simulink model "Torque Vectoring and Ackerman Model"  (R2020b)
settings: Solver=ode4  StartTime=0.0  StopTime=12  FixedStep=1e-5  RelTol=1e-3
InitFcn:
  | clc
  | clear
  | clc;
  | clear;
  | Ts=1e-5; %Sampling time
  | f=50; %Supply frequency
  | Rs=0.03553; %Stator resistance
  | Rr=0.02092; %Rotor resistance
  | Lls=0.000335; %Stator inductance
  | Llr=0.000335; %Rotor inductance
  | Lm=0.0151; %Mutual inductance
  | P=4; %Number of Poles
  | ts=(Lls+Lm)/Rs; % Stator time constant
  | Tr=(Llr+Lm)/Rr; % Rotor time constant
  | Ls=Lls+Lm;
  | Lrr=Llr+Lm;
  | J=1.25; %Inertia
  | F=0.03914; %Friction factor
  | VDC=580;
  | sigma=1-(Lm^2/(Ls*Lrr));
  | rs=Rs+Rr*(Lm/Lrr)^2;
  | Kp=1498*sigma*Ls;
  | Ki=rs*1498;
  | dw=1.55;
  | l=3;
  | m       =       1500;           %Vehicle mass
  | g       =       9.81;           %Gravitational acceleration
  | L       =          3;           %Distance between front axle and rear axle
  | Lf      =        1.3;           %Distance between center of mass and front axle
  | Lr      =       L-Lf;           %Distance between center of mass and rear axle
  | Cf      =      67369;           %Front track Cornering stiffness coef
  | Cr      =      63411;           %rear track Cornering stiffness coef
  | S       =        1.7;           %Area of frontal surface of the vehicle
  | CYB     =       -2.2;           %Force drag coef
  | CMzB    =        0.6;           %Moment drag coef
  | Mzfa    =       2010;           %Front track Aligning stiffness coef
  | Mzra    =       1366;           %rear track Aligning stiffness coef
  | rho     =      1.225;           %density
  | Iz      =       2000;           %Yaw Moment of Inertia
  | Kgear=1;
undefined symbols (not defined in the file): DiscIntNeverNeededParam, Driver, Wheels_Driver_VehDyn_Lib
libraries: pid_lib x12, powerlib_meascontrol x11, powerlib x9, simulink_extras x4
(part 1 of 2)
settings Model: Creator=Mostafa  LastModifiedBy=Mostafa

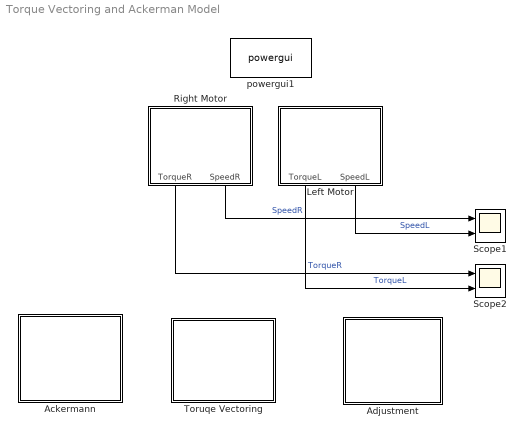
== system Torque Vectoring and Ackerman Model ==
  Ackermann : Subsystem
  Adjustment : Subsystem
  Left Motor : Subsystem
      settings: PortSchema="{\"entries\":[{\"content\":{\"sides\":[{\"content\":{\"connectorIds\":[]},\"type\":\"ConnectorPlacement.EquallySpacedRectSide\",\"uuid\":\"d60caa5e-c143-44b9-abe1-e5bc42f5c989\"},{\"content\":{\"connectorIds\":[],\"side\":\"RIGHT\"},\"type\":\"ConnectorPlacement.EquallySpacedRectSide\",\"uuid\":\"6d3ab839-fc24-43f3-9ba9-29c9b61bd22e\"},{\"content\":{\"connectorIds\":[],\"side\":\"TOP\"},\"type\":\"ConnectorPlacement.EquallySpacedRectSide\",\"uuid\":\"19f78343-3a34-4d8d-b4ff-ce8c56708ba0\"},{\"content\":{\"connectorIds\":[\"Out1\",\"Out2\"],\"side\":\"BOTTOM\"},\"type\":\"ConnectorPlacement.EquallySpacedRectSide\",\"uuid\":\"b455b762-473b-46a0-b917-5ab7203214ed\"},{\"content\":{\"connectorIds\":[],\"side\":\"HIDDEN\"},\"type\":\"ConnectorPlacement.EquallySpacedRectSide\",\"uuid\":\"ac9f86ca-680b-4222-bdb6-29216a90dea9\"}]},\"type\":\"ConnectorPlacement.EquallySpacedConnector\",\"uuid\":\"3823dedf-6920-4310-aeb6-55963e7ef5a8\"}],\"packageUris\":[\"http://schema.mathworks.com/mf0/Connector/R2020b\"],\"version\":\"1.0\"}"
      mask Display: image('D:\images.jpg'); % Use "Edit Image" on toolstrip to change.
  Right Motor : Subsystem
      settings: PortSchema="{\"entries\":[{\"content\":{\"sides\":[{\"content\":{\"connectorIds\":[]},\"type\":\"ConnectorPlacement.EquallySpacedRectSide\",\"uuid\":\"d60caa5e-c143-44b9-abe1-e5bc42f5c989\"},{\"content\":{\"connectorIds\":[],\"side\":\"RIGHT\"},\"type\":\"ConnectorPlacement.EquallySpacedRectSide\",\"uuid\":\"6d3ab839-fc24-43f3-9ba9-29c9b61bd22e\"},{\"content\":{\"connectorIds\":[],\"side\":\"TOP\"},\"type\":\"ConnectorPlacement.EquallySpacedRectSide\",\"uuid\":\"19f78343-3a34-4d8d-b4ff-ce8c56708ba0\"},{\"content\":{\"connectorIds\":[\"Out1\",\"Out2\"],\"side\":\"BOTTOM\"},\"type\":\"ConnectorPlacement.EquallySpacedRectSide\",\"uuid\":\"35fd2daf-de54-41dc-b20d-56980127e7c6\"},{\"content\":{\"connectorIds\":[],\"side\":\"HIDDEN\"},\"type\":\"ConnectorPlacement.EquallySpacedRectSide\",\"uuid\":\"ac9f86ca-680b-4222-bdb6-29216a90dea9\"}]},\"type\":\"ConnectorPlacement.EquallySpacedConnector\",\"uuid\":\"3823dedf-6920-4310-aeb6-55963e7ef5a8\"}],\"packageUris\":[\"http://schema.mathworks.com/mf0/Connector/R2020b\"],\"version\":\"1.0\"}"
      mask Display: image('D:\images.jpg'); % Use "Edit Image" on toolstrip to change.
  Scope1 : Scope  NumInputPorts=2
  Scope2 : Scope  NumInputPorts=2
  Toruqe Vectoring : Subsystem
  powergui1 : powerlib/powergui  Priority=1  SimulationMode=Continuous  SampleTime=1e-6  frequency=60  Iterations=50  frequencyindice=50  Pbase=100e6  ErrMax=1e-4  UnitsV=kV  UnitsW=MW  buscounter=0  FunctionMessages=off  echomessages=off  EnableUseOfTLC=off  CurrentSourceSwitches=off  DisableSnubberDevices=off  DisableRonSwitches=off  DisableVfSwitches=off  DisplayEquations=off  AutomaticDiscreteSolvers=off  SolverType=Tustin/Backward Euler (TBE)  Interpol=off  ExternalGateDelay=off  methode=off  Ts=100  x0status=blocks  SPID=on  SwTol=0  HookPort=off  NonlinearTolerance=1e-4  nMaxIteration=100  ContinueOnMaxIteration=off  RestoreLinks=warning  ResistiveCurrentMeasurement=off  Frange=[0:2:500]  Ylog=off  Xlog=on  ShowGrid=off  save=off  variable=ZData  structure=0  ZoomFFT=off  StartTime=0.0  cycles=1  DisplayStyle=1  fundamental=60  FreqAxis=off  MaxFrequency=1000  frequencyindicesteady=1  RmsSteady=1  display=off
  wires:
  Right Motor/2(SpeedR) -> Scope1/1  "SpeedR"
  Left Motor/2(SpeedL) -> Scope1/2  "SpeedL"
  Right Motor/1(TorqueR) -> Scope2/1  "TorqueR"
  Left Motor/1("TorqueL ") -> Scope2/2  "TorqueL"

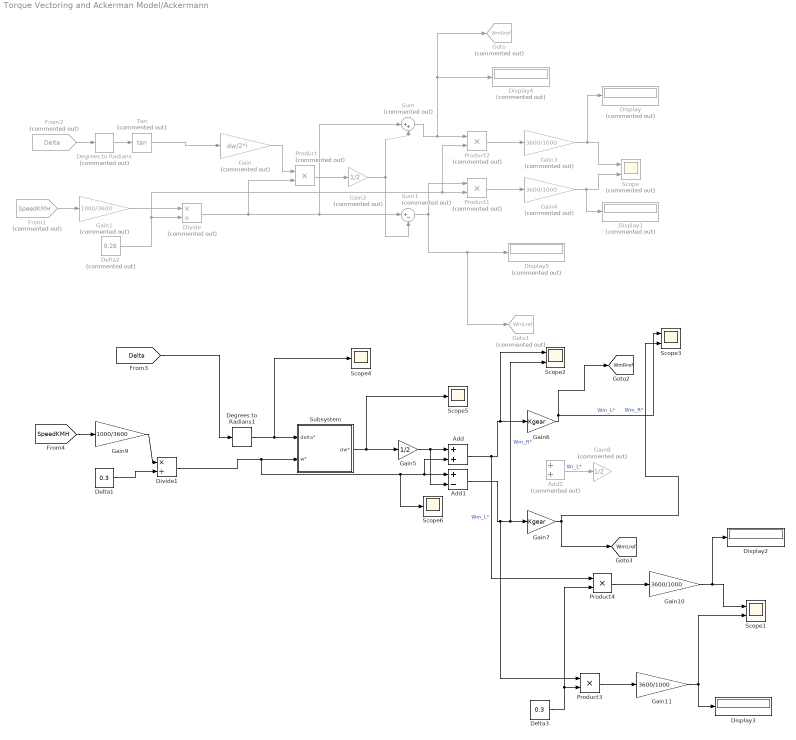
== system Torque Vectoring and Ackerman Model/Ackermann ==
  Add : Sum
  Add1 : Sum  Inputs=+-
  Add2 : Sum  Commented=on
  Degrees to Radians : simulink_extras/Transformations/Degrees to Radians  Commented=on
  Degrees to Radians1 : simulink_extras/Transformations/Degrees to Radians
  Delta1 : Constant  Value=0.3
  Delta2 : Constant  Commented=on  Value=0.26
  Delta3 : Constant  Value=0.3
  Display{,1,4..5} (4 alike) : Display  Commented=on
  Display2 : Display
  Display3 : Display
  Divide : Product  Commented=on  Inputs=*/
  Divide1 : Product  Inputs=*/
  From1 : From  Commented=on  GotoTag=SpeedKMH  TagVisibility=global
  From2 : From  Commented=on  GotoTag=Delta  TagVisibility=global
  Gain : Gain  Commented=on  Gain=dw/2*l
  Gain1 : Gain  Commented=on  Gain=1000/3600
  Gain10 : Gain  Gain=3600/1000
  Gain11 : Gain  Gain=3600/1000
  Gain2 : Gain  Commented=on  Gain=1/2
  Gain3 : Gain  Commented=on  Gain=3600/1000
  Gain4 : Gain  Commented=on  Gain=3600/1000
  Gain5 : Gain  Gain=1/2
  Gain6 : Gain  Gain=Kgear
  Gain7 : Gain  Gain=Kgear
  Gain8 : Gain  Commented=on  Gain=1/2
  Gain9 : Gain  Gain=1000/3600
  Goto : Goto  Commented=on  GotoTag=WmRref  TagVisibility=global
  Goto1 : Goto  Commented=on  GotoTag=WmLref  TagVisibility=global
  Product : Product  Commented=on
  Product1 : Product  Commented=on
  Product2 : Product  Commented=on
  Product3 : Product
  Product4 : Product
  Scope : Scope  Commented=on  NumInputPorts=2
  Scope1 : Scope  NumInputPorts=2
  Scope2 : Scope  NumInputPorts=2
  Scope3 : Scope  NumInputPorts=2
  Scope4 : Scope
  Scope5 : Scope
  Scope6 : Scope
  Subsystem : Subsystem
  Sum : Sum  Commented=on  Inputs=|++
  Sum1 : Sum  Commented=on  Inputs=|+-
  Tan : Trigonometry  Commented=on  Operator=tan
  tag scope: WmLref=global, WmRref=global
  wires:
  Degrees to Radians/1 -> Tan/1
  Tan/1 -> Gain/1
  Gain/1 -> Product/1
  Product/1 -> Gain2/1
  Gain2/1 -> Sum1/2, Sum/2
  Divide/1 -> Product/2, Sum/1, Sum1/1
  Gain1/1 -> Divide/1
  Sum1/1 -> Product1/1, Goto1/1, Display5/1
  Delta2/1 -> Product2/2, Product1/2, Divide/2
  Product2/1 -> Gain3/1
  Product1/1 -> Gain4/1
  Gain4/1 -> Display1/1, Scope/2
  Gain3/1 -> Display/1, Scope/1
  Sum/1 -> Display4/1, Goto/1, Product2/1
  From1/1 -> Gain1/1
  From2/1 -> Degrees to Radians/1
  Degrees to Radians1/1 -> Scope4/1, Subsystem/1(delta*)
  Gain5/1 -> Add1/2, Add/1
  Gain6/1 -> Scope3/1, [WmRref]  "Wm_L*"
  Subsystem/1(dw*) -> Scope5/1, Gain5/1
  Add2/1 -> Gain8/1  "Wr_L*"
  Gain7/1 -> Scope3/2, [WmLref]  "Wm_R*"
  Gain9/1 -> Divide1/1
  [SpeedKMH] -> Gain9/1
  Delta1/1 -> Divide1/2
  [Delta] -> Degrees to Radians1/1
  Divide1/1 -> Scope6/1, Add/2, Add1/1, Subsystem/2(w*)
  Delta3/1 -> Product4/2, Product3/2
  Gain10/1 -> Scope1/1, Display2/1
  Product4/1 -> Gain10/1
  Gain11/1 -> Scope1/2, Display3/1
  Add/1 -> Product4/1, Scope2/1, Gain6/1  "Wm_L*"
  Add1/1 -> Product3/1, Scope2/2, Gain7/1  "Wm_R*"
  Product3/1 -> Gain11/1

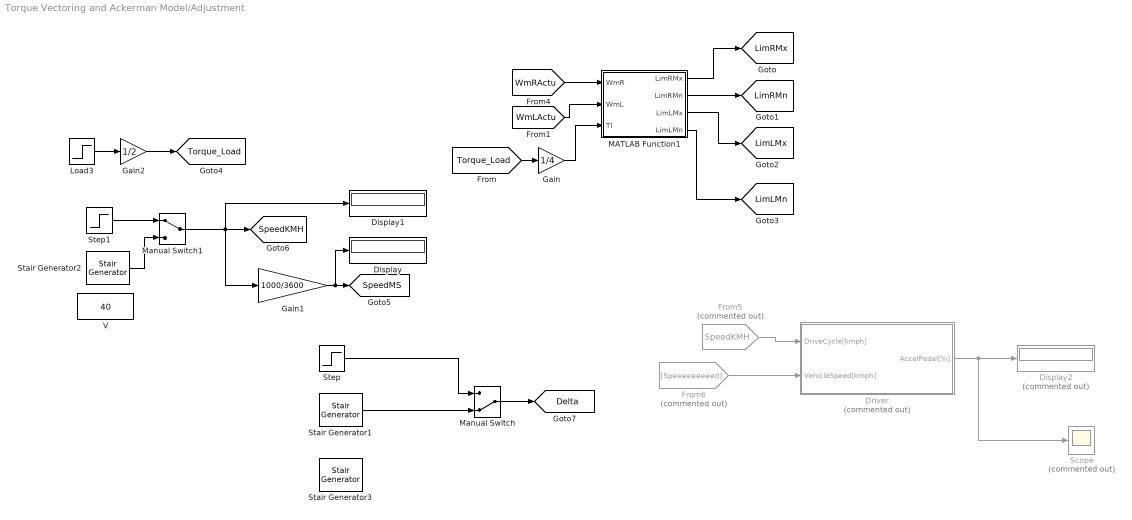
== system Torque Vectoring and Ackerman Model/Adjustment ==
  Display : Display
  Display1 : Display
  Display2 : Display  Commented=on
  Driver : Subsystem  Commented=on  AncestorBlock=Wheels_Driver_VehDyn_Lib/Driver
  From5 : From  Commented=on  GotoTag=SpeedKMH  TagVisibility=global
  From6 : From  Commented=on  GotoTag=Speeeeeeeeed  TagVisibility=global
  Gain : Gain  Gain=1/4
  Gain1 : Gain  Gain=1000/3600
  Gain2 : Gain  Gain=1/2
  Load3 : Step  Time=3  After=800  SampleTime=Ts
  MATLAB Function1 : MATLAB Function  TreatAsAtomicUnit=on
  Manual Switch : ManualSwitch  CurrentSetting=0
  Manual Switch1 : ManualSwitch
  Scope : Scope  Commented=on
  Stair Generator1 : powerlib_meascontrol/Pulse & Signal Generators/Stair Generator  t="[0 4 6 8 10  ]"  e=[0 10 0 -10 0 ]  Ts=0
  Stair Generator2 : powerlib_meascontrol/Pulse & Signal Generators/Stair Generator  t=[0 3 5 7 9 10 ]  e=[0 50 100 -50 -100 0 ]  Ts=0
  Stair Generator3 : powerlib_meascontrol/Pulse & Signal Generators/Stair Generator  t=[0 3 5 7 9 10 ]  e=[0 5 10 -5 10 0 ]  Ts=0
  Step : Step  Time=4  After=10  SampleTime=0
  Step1 : Step  Time=3  After=36  SampleTime=0
  V : Constant  Value=40
  tag scope: Delta=global, LimLMn=global, LimLMx=global, LimRMn=global, LimRMx=global, SpeedKMH=global, SpeedMS=global, Torque_Load=global
  wires:
  Gain1/1 -> Display/1, [SpeedMS]
  Load3/1 -> Gain2/1
  Step/1 -> Manual Switch/1
  Manual Switch/1 -> [Delta]
  Stair Generator1/1 -> Manual Switch/2
  [WmRActu] -> MATLAB Function1/1(WmR)
  [WmLActu] -> MATLAB Function1/2(WmL)
  MATLAB Function1/3(LimLMx) -> [LimLMx]
  MATLAB Function1/4(LimLMn) -> [LimLMn]
  MATLAB Function1/1(LimRMx) -> [LimRMx]
  MATLAB Function1/2(LimRMn) -> [LimRMn]
  Manual Switch1/1 -> Gain1/1, Display1/1, [SpeedKMH]
  Step1/1 -> Manual Switch1/1
  Stair Generator2/1 -> Manual Switch1/2
  [Torque_Load] -> Gain/1
  Gain/1 -> MATLAB Function1/3(Tl)
  From5/1 -> Driver/1(" DriveCycle[kmph]")
  From6/1 -> Driver/2(VehicleSpeed[kmph])
  Driver/1(AccelPedal[%]) -> Scope/1, Display2/1
  Gain2/1 -> [Torque_Load]

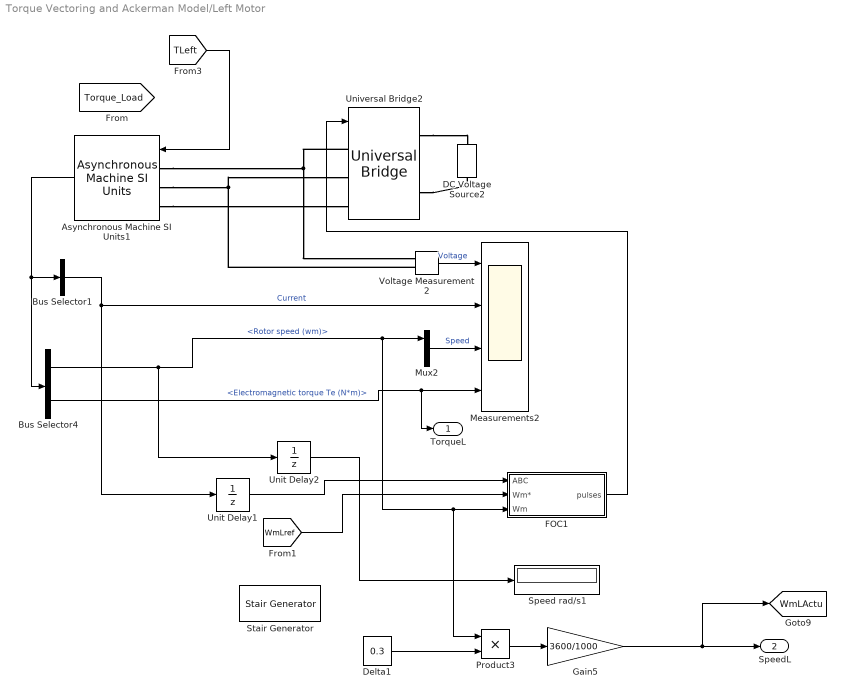
== system Torque Vectoring and Ackerman Model/Left Motor ==
  Asynchronous Machine SI Units1 : powerlib/Machines/Asynchronous Machine SI Units  RotorType=Squirrel-cage  PresetModel="19:  100 HP (75KW)  400 V 50Hz 1484 RPM"  MechanicalLoad=Torque Tm  ShowDetailedParameters=on  ReferenceFrame=Rotor  Units=SI  MeasurementBus=off  NominalParameters=[7.5e+04 400 50]  Stator=[0.03552 0.000335]  Rotor=[0.02092 0.000335]  Cage1=[0.4155 0.002066]  Cage2=[0.4168 0.0003495]  Lm=0.0151  Mechanical=[1.25 0.03914 2]  PolePairs=2  InitialConditions=[1 0 0 0 0 0 0 0]  SimulateSaturation=off  Saturation=[14.03593122, 27.81365428, 53.79336849, 72.68890987, 97.98006896, 148.6815601, 215.7428561, 302.9841135, 428.7778367 ; 230, 322, 414, 460, 506, 552, 598, 644, 690]  LoadFlowParameters=1492000  TsPowergui=0  TsBlock=-1  IterativeModel=Trapezoidal non iterative  IterativeDiscreteModel=Trapezoidal non iterative  Pmec=1.492e+006
  Bus Selector1 : BusSelector  OutputSignals=Stator measurements.Stator current is_a (A),Stator measurements.Stator current is_b (A),Stator measurements.Stator current is_c (A)  OutputAsBus=on
  Bus Selector4 : BusSelector  OutputSignals=Mechanical.Rotor speed (wm),Mechanical.Electromagnetic torque Te (N*m)
  DC Voltage Source2 : powerlib/Electrical Sources/DC Voltage Source  Amplitude=VDC  Measurements=None
  Delta1 : Constant  Value=0.3
  FOC1 : Subsystem
  Gain5 : Gain  Gain=3600/1000
  Measurements2 : Scope  NumInputPorts=4
  Mux2 : Mux  Inputs=2
  Product3 : Product
  Speed rad/s1 : Display
  Stair Generator : powerlib_meascontrol/Pulse & Signal Generators/Stair Generator  t=[0 2 3 4 5 6 ]  e=[0 95 60 105 70 -120 ]  Ts=Ts
  Unit Delay1 : UnitDelay  SampleTime=-1  HasFrameUpgradeWarning=on
  Unit Delay2 : UnitDelay  SampleTime=-1  HasFrameUpgradeWarning=on
  Universal Bridge2 : powerlib/Power Electronics/Universal Bridge  Arms=3  SnubberResistance=1e5  SnubberCapacitance=inf  Device=IGBT / Diodes  Ron=1e-3  Lon=0  ForwardVoltages="[  0  0  ]"  ForwardVoltage=0  GTOparameters=[ 10e-6 , 20e-6 ]  IGBTparameters=[ 1e-6 , 2e-6 ]  Measurements=None  Measurements_2=None  converterType=Rectifier
  Voltage Measurement2 : powerlib/Measurements/Voltage Measurement  PhasorSimulation=off  OutputType=Complex  PSBequivalent=0
  "TorqueL " : Outport
  SpeedL : Outport  Port=2
  tag scope: WmLActu=global
  wires:
  Voltage Measurement2/1 -> Measurements2/1  "Voltage"
  Asynchronous Machine SI Units1/1 -> Bus Selector1/1, Bus Selector4/1
  Bus Selector1/1 -> Measurements2/2, Unit Delay1/1  "Current"
  Bus Selector4/1 -> Unit Delay2/1, Mux2/1, Product3/1, FOC1/3(Wm)  "<Rotor speed (wm)>"
  Unit Delay2/1 -> Speed rad/s1/1
  Bus Selector4/2 -> "TorqueL "/1, Measurements2/4  "<Electromagnetic torque Te (N*m)>"
  Mux2/1 -> Measurements2/3  "Speed"
  Unit Delay1/1 -> FOC1/1(ABC)
  FOC1/1(pulses) -> Universal Bridge2/1
  Delta1/1 -> Product3/2
  Product3/1 -> Gain5/1
  [WmLref] -> FOC1/2(Wm*)
  [TLeft] -> Asynchronous Machine SI Units1/1
  Gain5/1 -> [WmLActu], SpeedL/1
  connections:
  Universal Bridge2/RConn2 -- DC Voltage Source2/LConn1
  Universal Bridge2/RConn1 -- DC Voltage Source2/RConn1
  Asynchronous Machine SI Units1/LConn3 -- Universal Bridge2/LConn3
  Voltage Measurement2/LConn2 -- Universal Bridge2/LConn2 -- Asynchronous Machine SI Units1/LConn2
  Universal Bridge2/LConn1 -- Voltage Measurement2/LConn1 -- Asynchronous Machine SI Units1/LConn1

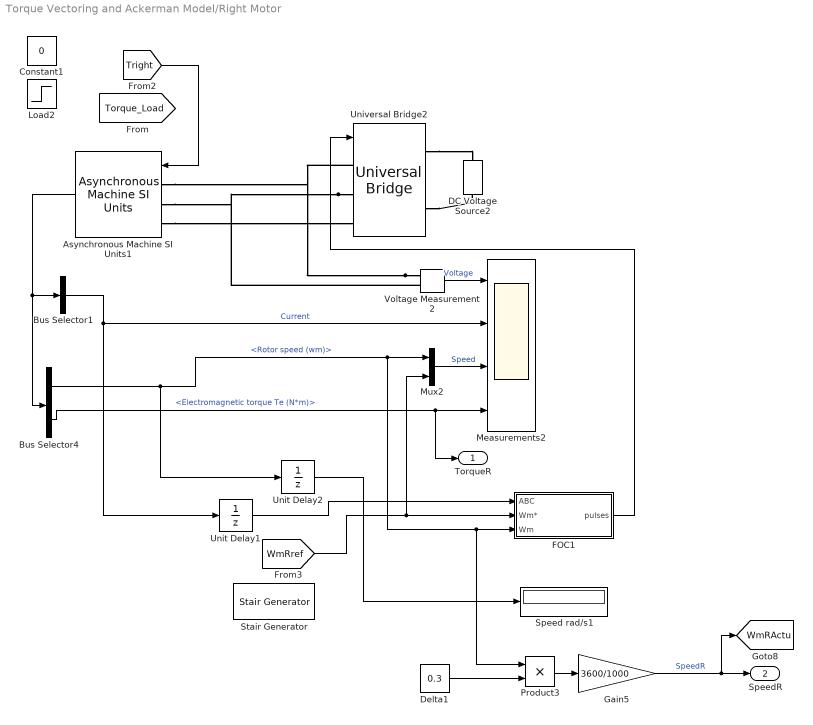
== system Torque Vectoring and Ackerman Model/Right Motor ==
  Asynchronous Machine SI Units1 : powerlib/Machines/Asynchronous Machine SI Units  RotorType=Squirrel-cage  PresetModel="19:  100 HP (75KW)  400 V 50Hz 1484 RPM"  MechanicalLoad=Torque Tm  ShowDetailedParameters=on  ReferenceFrame=Rotor  Units=SI  MeasurementBus=off  NominalParameters=[7.5e+04 400 50]  Stator=[0.03552 0.000335]  Rotor=[0.02092 0.000335]  Cage1=[0.4155 0.002066]  Cage2=[0.4168 0.0003495]  Lm=0.0151  Mechanical=[1.25 0.03914 2]  PolePairs=2  InitialConditions=[1 0 0 0 0 0 0 0]  SimulateSaturation=off  Saturation=[14.03593122, 27.81365428, 53.79336849, 72.68890987, 97.98006896, 148.6815601, 215.7428561, 302.9841135, 428.7778367 ; 230, 322, 414, 460, 506, 552, 598, 644, 690]  LoadFlowParameters=1492000  TsPowergui=0  TsBlock=-1  IterativeModel=Trapezoidal non iterative  IterativeDiscreteModel=Trapezoidal non iterative  Pmec=1.492e+006
  Bus Selector1 : BusSelector  OutputSignals=Stator measurements.Stator current is_a (A),Stator measurements.Stator current is_b (A),Stator measurements.Stator current is_c (A)  OutputAsBus=on
  Bus Selector4 : BusSelector  OutputSignals=Mechanical.Rotor speed (wm),Mechanical.Electromagnetic torque Te (N*m)
  Constant1 : Constant  Value=0
  DC Voltage Source2 : powerlib/Electrical Sources/DC Voltage Source  Amplitude=VDC  Measurements=None
  Delta1 : Constant  Value=0.3
  FOC1 : Subsystem
  Gain5 : Gain  Gain=3600/1000
  Load2 : Step  Time=0.5  After=3  SampleTime=Ts
  Measurements2 : Scope  NumInputPorts=4
  Mux2 : Mux  Inputs=2
  Product3 : Product
  Speed rad/s1 : Display
  Stair Generator : powerlib_meascontrol/Pulse & Signal Generators/Stair Generator  t=[0 2 3 4 5 6 ]  e=[0 95 60 105 70 -120 ]  Ts=Ts
  Unit Delay1 : UnitDelay  SampleTime=-1  HasFrameUpgradeWarning=on
  Unit Delay2 : UnitDelay  SampleTime=-1  HasFrameUpgradeWarning=on
  Universal Bridge2 : powerlib/Power Electronics/Universal Bridge  Arms=3  SnubberResistance=1e5  SnubberCapacitance=inf  Device=IGBT / Diodes  Ron=1e-3  Lon=0  ForwardVoltages="[  0  0  ]"  ForwardVoltage=0  GTOparameters=[ 10e-6 , 20e-6 ]  IGBTparameters=[ 1e-6 , 2e-6 ]  Measurements=None  Measurements_2=None  converterType=Rectifier
  Voltage Measurement2 : powerlib/Measurements/Voltage Measurement  PhasorSimulation=off  OutputType=Complex  PSBequivalent=0
  TorqueR : Outport
  SpeedR : Outport  Port=2
  tag scope: WmRActu=global
  wires:
  FOC1/1(pulses) -> Universal Bridge2/1
  Unit Delay1/1 -> FOC1/1(ABC)
  Mux2/1 -> Measurements2/3  "Speed"
  Bus Selector4/2 -> TorqueR/1, Measurements2/4  "<Electromagnetic torque Te (N*m)>"
  Unit Delay2/1 -> Speed rad/s1/1
  Bus Selector4/1 -> Product3/1, FOC1/3(Wm), Mux2/1, Unit Delay2/1  "<Rotor speed (wm)>"
  Bus Selector1/1 -> Unit Delay1/1, Measurements2/2  "Current"
  Asynchronous Machine SI Units1/1 -> Bus Selector4/1, Bus Selector1/1
  Voltage Measurement2/1 -> Measurements2/1  "Voltage"
  Delta1/1 -> Product3/2
  Gain5/1 -> [WmRActu], SpeedR/1  "SpeedR"
  Product3/1 -> Gain5/1
  [WmRref] -> Mux2/2, FOC1/2(Wm*)
  [Tright] -> Asynchronous Machine SI Units1/1
  connections:
  Voltage Measurement2/LConn1 -- Universal Bridge2/LConn1 -- Asynchronous Machine SI Units1/LConn1
  Universal Bridge2/LConn2 -- Voltage Measurement2/LConn2 -- Asynchronous Machine SI Units1/LConn2
  Asynchronous Machine SI Units1/LConn3 -- Universal Bridge2/LConn3
  Universal Bridge2/RConn1 -- DC Voltage Source2/RConn1
  Universal Bridge2/RConn2 -- DC Voltage Source2/LConn1

== system Torque Vectoring and Ackerman Model/Toruqe Vectoring ==
  CorrectionModel : Subsystem
  KinematicModel : Subsystem
  Scope : Scope
  Scope1 : Scope
  tag scope: Yawrate=global, beta=global
  wires:
  KinematicModel/1(SideSlip) -> [beta], Scope/1
  [SpeedMS] -> CorrectionModel/1(speed), KinematicModel/1(speed)
  KinematicModel/2(YawRate) -> Scope1/1, [Yawrate]
  [Delta] -> KinematicModel/2(Delta), CorrectionModel/2(Delta)

== system Torque Vectoring and Ackerman Model/Ackermann/Subsystem ==
  delta* : Inport
  w* : Inport  Port=2
  Constant : Constant  Value=dw
  Constant1 : Constant  Value=l
  Divide : Product  Inputs=**
  Divide1 : Product  Inputs=*/
  Divide2 : Product  Inputs=**
  Tan : Trigonometry  Operator=tan
  dw* : Outport
  wires:
  delta*/1 -> Tan/1
  Tan/1 -> Divide/1
  Constant/1 -> Divide/2
  Divide/1 -> Divide1/1
  Constant1/1 -> Divide1/2
  Divide1/1 -> Divide2/1
  w*/1 -> Divide2/2
  Divide2/1 -> dw*/1

== system Torque Vectoring and Ackerman Model/Adjustment/Driver ==
  " DriveCycle[kmph]" : Inport
  VehicleSpeed[kmph] : Inport  Port=2
  APPDynamics : TransferFcn  Denominator=[0.1 1]
  Accel : Saturate  UpperLimit=100  LowerLimit=0
  PID Controller : pid_lib/PID Controller  Controller=PI  Form=Parallel  TimeDomain=Continuous-time  UseExternalTs=off  SampleTime=-1  IntegratorMethod=Forward Euler  FilterMethod=Forward Euler  ControllerParametersSource=internal  P=20  I=1  D=0  UseFilter=on  N=100  TunerSelectOption=Transfer Function Based (PID Tuner App)  InitialConditionSource=internal  InitialConditionForIntegrator=0  InitialConditionForFilter=0  DifferentiatorICPrevScaledInput=0  ExternalReset=none  TrackingMode=off  Kt=1  LimitOutput=on  SatLimitsSource=internal  UpperSaturationLimit=100  LowerSaturationLimit=-100  LinearizeAsGain=on  AntiWindupMode=none  Kb=1  POutMin=[]  POutMax=[]  IOutMin=[]  IOutMax=[]  DOutMin=[]  DOutMax=[]  NOutMin=[]  NOutMax=[]  SumOutMin=[]  SumOutMax=[]  SaturationOutMin=[]  SaturationOutMax=[]  PParamMin=[]  PParamMax=[]  IParamMin=[]  IParamMax=[]  DParamMin=[]  DParamMax=[]  NParamMin=[]  NParamMax=[]  KbParamMin=[]  KbParamMax=[]  KtParamMin=[]  KtParamMax=[]  KbOutMin=[]  KbOutMax=[]  KtOutMin=[]  KtOutMax=[]  IntegratorOutMin=[]  IntegratorOutMax=[]  FilterOutMin=[]  FilterOutMax=[]  SumI1OutMin=[]  SumI1OutMax=[]  SumI2OutMin=[]  SumI2OutMax=[]  SumI3OutMin=[]  SumI3OutMax=[]  SumI4OutMin=[]  SumI4OutMax=[]  SumDOutMin=[]  SumDOutMax=[]  DifferentiatorOutMin=[]  DifferentiatorOutMax=[]  FilterDiffOutCoefMin=[]  FilterDiffOutCoefMax=[]  ReciprocalOutMin=[]  ReciprocalOutMax=[]  SumDenOutMin=[]  SumDenOutMax=[]  SumNumOutMin=[]  SumNumOutMax=[]  DivideOutMin=[]  DivideOutMax=[]  UdiffTsProdOutMin=[]  UdiffTsProdOutMax=[]  NTsProdOutMin=[]  NTsProdOutMax=[]  UintegralTsProdOutMin=[]  UintegralTsProdOutMax=[]  UngainTsProdOutMin=[]  UngainTsProdOutMax=[]  IntegratorContinuousStateAttributes=''  IntegratorStateMustResolveToSignalObject=off  IntegratorRTWStateStorageClass=Auto  FilterContinuousStateAttributes=''  FilterStateMustResolveToSignalObject=off  FilterRTWStateStorageClass=Auto  ParallelPVariant=InternalParameters  IdealPVariant=Disabled  IVariant=InternalParameters  DVariant=Disabled  IntegratorVariant=Continuous  SatVariant=Enabled  AWVariant=Passthrough  PCopyVariant=Disabled  TRVariant=Disabled  FdbkBlocksVariant=Forward  IdealPFdbkVariant=Disabled  SatFdbkVariant=Disabled  DerivativeFilterVariant=Disabled  NVariant=Disabled  NCopyVariant=Disabled_SignalSpec  FilterICVariant=Disabled  IntegratorICVariant=InternalICs  ExternalResetVariant=Disabled  TRSumVariant=Passthrough  SumFdbkVariant=Disabled  SumVariant=Sum_PI  TsampFilterVariant=InternalTs  TsampNgainVariant=Passthrough  TsampIntegralVariant=Passthrough  ExternalSaturationOutDataTypeStr=Inherit: Same as second input
  Sum : Sum  Inputs=|+-
  AccelPedal[%] : Outport  VectorParamsAs1DForOutWhenUnconnected=off
  wires:
  " DriveCycle[kmph]"/1 -> Sum/1
  VehicleSpeed[kmph]/1 -> Sum/2
  PID Controller/1 -> Accel/1
  Sum/1 -> PID Controller/1
  Accel/1 -> APPDynamics/1
  APPDynamics/1 -> AccelPedal[%]/1

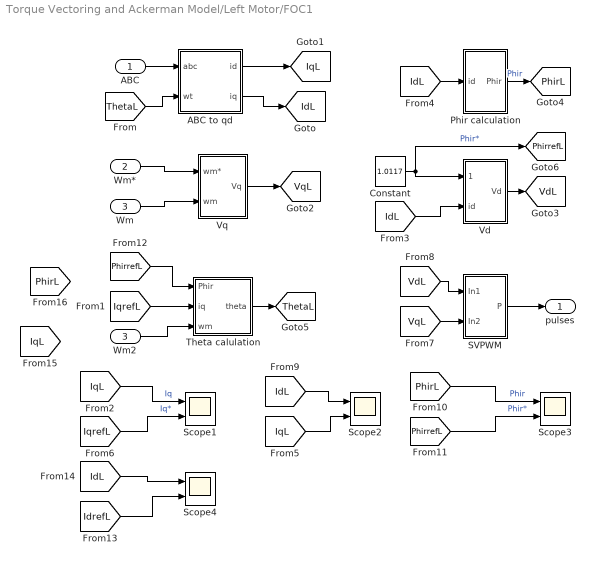
== system Torque Vectoring and Ackerman Model/Left Motor/FOC1 ==
  ABC : Inport
  Wm* : Inport  Port=2
  Wm : Inport  Port=3
  ABC to qd : Subsystem
  Constant : Constant  Value=1.0117
  Phir calculation : Subsystem
  SVPWM : Subsystem
  Scope{1..4} (4 alike) : Scope  NumInputPorts=2
  Theta calulation : Subsystem
  Vd : Subsystem
  Vq : Subsystem
  Wm2 : InportShadow  Port=3
  pulses : Outport
  tag scope: IdL=global, IqL=global, PhirL=global, PhirrefL=global, ThetaL=global, VdL=global, VqL=global
  wires:
  [IqrefL] -> Theta calulation/2(iq)
  [PhirrefL] -> Theta calulation/1(Phir)
  [IdrefL] -> Scope4/2
  [IdL] -> Scope4/1
  [PhirL] -> Scope3/1  "Phir"
  [PhirrefL] -> Scope3/2  "Phir*"
  [IdL] -> Scope2/1
  [IqL] -> Scope2/2
  [IqrefL] -> Scope1/2  "Iq*"
  [IqL] -> Scope1/1  "Iq"
  Vd/1(Vd) -> [VdL]
  [IdL] -> Vd/2(id)
  Constant/1 -> [PhirrefL], Vd/1(Phir*)  "Phir*"
  Theta calulation/1(theta) -> [ThetaL]
  Wm2/1 -> Theta calulation/3(wm)
  SVPWM/1(P) -> pulses/1
  [VqL] -> SVPWM/2(In2)
  [VdL] -> SVPWM/1(In1)
  Phir calculation/1(Phir) -> [PhirL]  "Phir"
  [IdL] -> Phir calculation/1(id)
  ABC to qd/2(iq) -> [IdL]
  ABC to qd/1(id) -> [IqL]
  [ThetaL] -> ABC to qd/2(wt)
  ABC/1 -> ABC to qd/1(abc)
  Vq/1(Vq) -> [VqL]
  Wm/1 -> Vq/2(wm)
  Wm*/1 -> Vq/1(wm*)

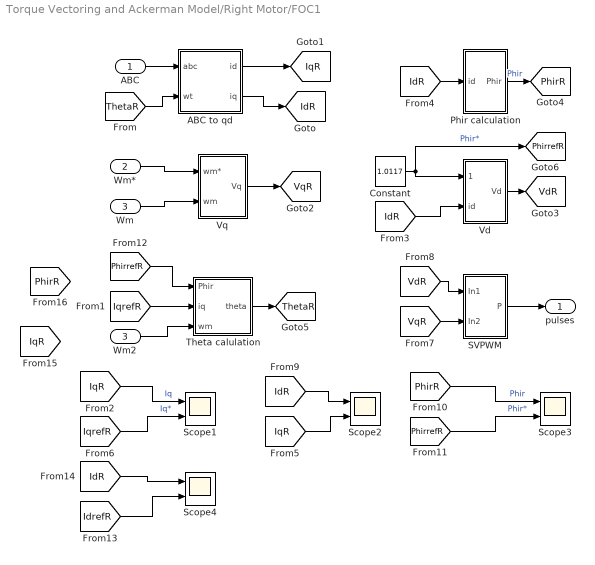
== system Torque Vectoring and Ackerman Model/Right Motor/FOC1 ==
  ABC : Inport
  Wm* : Inport  Port=2
  Wm : Inport  Port=3
  ABC to qd : Subsystem
  Constant : Constant  Value=1.0117
  Phir calculation : Subsystem
  SVPWM : Subsystem
  Scope{1..4} (4 alike) : Scope  NumInputPorts=2
  Theta calulation : Subsystem
  Vd : Subsystem
  Vq : Subsystem
  Wm2 : InportShadow  Port=3
  pulses : Outport
  tag scope: IdR=global, IqR=global, PhirR=global, PhirrefR=global, ThetaR=global, VdR=global, VqR=global
  wires:
  Wm*/1 -> Vq/1(wm*)
  Wm/1 -> Vq/2(wm)
  Vq/1(Vq) -> [VqR]
  ABC/1 -> ABC to qd/1(abc)
  [ThetaR] -> ABC to qd/2(wt)
  ABC to qd/1(id) -> [IqR]
  ABC to qd/2(iq) -> [IdR]
  [IdR] -> Phir calculation/1(id)
  Phir calculation/1(Phir) -> [PhirR]  "Phir"
  [VdR] -> SVPWM/1(In1)
  [VqR] -> SVPWM/2(In2)
  SVPWM/1(P) -> pulses/1
  Wm2/1 -> Theta calulation/3(wm)
  Theta calulation/1(theta) -> [ThetaR]
  Constant/1 -> Vd/1(Phir*), [PhirrefR]  "Phir*"
  [IdR] -> Vd/2(id)
  Vd/1(Vd) -> [VdR]
  [IqR] -> Scope1/1  "Iq"
  [IqrefR] -> Scope1/2  "Iq*"
  [IqR] -> Scope2/2
  [IdR] -> Scope2/1
  [PhirrefR] -> Scope3/2  "Phir*"
  [PhirR] -> Scope3/1  "Phir"
  [IdR] -> Scope4/1
  [IdrefR] -> Scope4/2
  [PhirrefR] -> Theta calulation/1(Phir)
  [IqrefR] -> Theta calulation/2(iq)

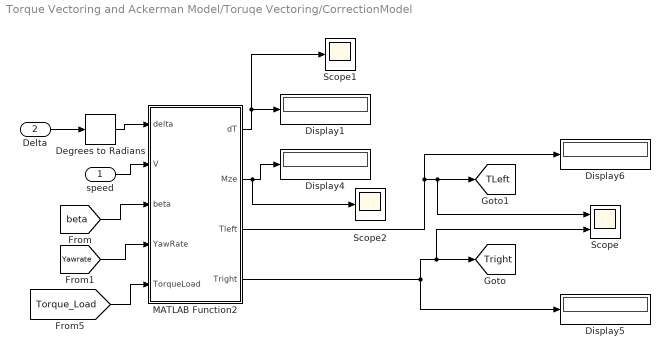
== system Torque Vectoring and Ackerman Model/Toruqe Vectoring/CorrectionModel ==
  speed : Inport
  Delta : Inport  Port=2
  Degrees to Radians : simulink_extras/Transformations/Degrees to Radians
  Display{1,4..6} (4 alike) : Display
  MATLAB Function2 : MATLAB Function  TreatAsAtomicUnit=on
  Scope : Scope  NumInputPorts=2
  Scope1 : Scope
  Scope2 : Scope
  tag scope: TLeft=global, Tright=global
  wires:
  Degrees to Radians/1 -> MATLAB Function2/1(delta)
  Delta/1 -> Degrees to Radians/1
  speed/1 -> MATLAB Function2/2(V)
  MATLAB Function2/2(Mze) -> Scope2/1, Display4/1
  [beta] -> MATLAB Function2/3(beta)
  [Yawrate] -> MATLAB Function2/4(YawRate)
  MATLAB Function2/4(Tright) -> Scope/2, [Tright], Display5/1
  MATLAB Function2/3(Tleft) -> Display6/1, Scope/1, [TLeft]
  [Torque_Load] -> MATLAB Function2/5(TorqueLoad)
  MATLAB Function2/1(dT) -> Scope1/1, Display1/1

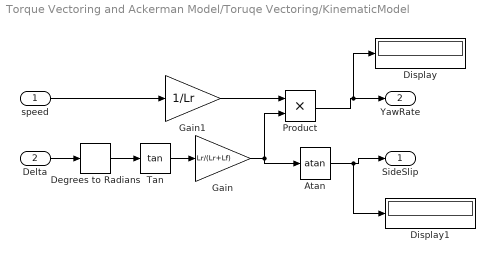
== system Torque Vectoring and Ackerman Model/Toruqe Vectoring/KinematicModel ==
  speed : Inport
  Delta : Inport  Port=2
  Atan : Trigonometry  Operator=atan
  Degrees to Radians : simulink_extras/Transformations/Degrees to Radians
  Display : Display
  Display1 : Display
  Gain : Gain  Gain=Lr/(Lr+Lf)
  Gain1 : Gain  Gain=1/Lr
  Product : Product
  Tan : Trigonometry  Operator=tan
  SideSlip : Outport
  YawRate : Outport  Port=2
  wires:
  Delta/1 -> Degrees to Radians/1
  Tan/1 -> Gain/1
  Atan/1 -> Display1/1, SideSlip/1
  Gain/1 -> Product/2, Atan/1
  speed/1 -> Gain1/1
  Gain1/1 -> Product/1
  Product/1 -> Display/1, YawRate/1
  Degrees to Radians/1 -> Tan/1

== system Torque Vectoring and Ackerman Model/Left Motor/FOC1/ABC to qd ==
  abc : Inport
  wt : Inport  Port=2
  Demux : Demux  Outputs=3
  Terminator : Terminator
  Unit Delay : UnitDelay  SampleTime=-1  HasFrameUpgradeWarning=on
  Unit Delay1 : UnitDelay  SampleTime=-1  HasFrameUpgradeWarning=on
  abc to dq0 : powerlib_meascontrol/Transformations/abc to dq0  Alignment=90 degrees behind phase A axis
  id : Outport
  iq : Outport  Port=2
  wires:
  abc/1 -> abc to dq0/1
  Unit Delay1/1 -> id/1
  wt/1 -> abc to dq0/2
  Unit Delay/1 -> iq/1
  Demux/2 -> Unit Delay1/1
  abc to dq0/1 -> Demux/1
  Demux/3 -> Terminator/1
  Demux/1 -> Unit Delay/1

== system Torque Vectoring and Ackerman Model/Left Motor/FOC1/Phir calculation ==
  id : Inport
  Transfer Fcn : TransferFcn  Numerator=[Lm]  Denominator=[Tr 1]
  Phir : Outport
  wires:
  id/1 -> Transfer Fcn/1
  Transfer Fcn/1 -> Phir/1

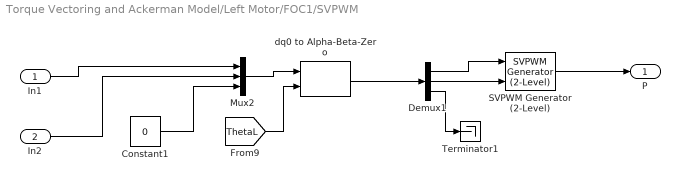
== system Torque Vectoring and Ackerman Model/Left Motor/FOC1/SVPWM ==
  In1 : Inport
  In2 : Inport  Port=2
  Constant1 : Constant  Value=0
  Demux1 : Demux  Outputs=3
  Mux2 : Mux  Inputs=3
  SVPWM Generator (2-Level) : powerlib_meascontrol/Pulse & Signal Generators/SVPWM Generator (2-Level)  InputType=alpha-beta components  SwitchingPattern=Pattern #1  Fc=5000  ParUref=[0.8 -30 50]  Ts=0
      settings: SourceProductBaseCode=PS
  Terminator1 : Terminator
  dq0 to Alpha-Beta-Zero : powerlib_meascontrol/Transformations/dq0 to Alpha-Beta-Zero  Alignment=90 degrees behind phase A axis
      settings: SourceProductBaseCode=PS
  P : Outport
  wires:
  Demux1/1 -> SVPWM Generator (2-Level)/1
  Constant1/1 -> Mux2/3
  dq0 to Alpha-Beta-Zero/1 -> Demux1/1
  [ThetaL] -> dq0 to Alpha-Beta-Zero/2
  In2/1 -> Mux2/2
  SVPWM Generator (2-Level)/1 -> P/1
  In1/1 -> Mux2/1
  Mux2/1 -> dq0 to Alpha-Beta-Zero/1
  Demux1/3 -> Terminator1/1
  Demux1/2 -> SVPWM Generator (2-Level)/2

== system Torque Vectoring and Ackerman Model/Left Motor/FOC1/Theta calulation ==
  Phir : Inport
  iq : Inport  Port=2
  wm : Inport  Port=3
  Add : Sum
  Discrete-Time Integrator : DiscreteIntegrator  SampleTime=Ts  ICPrevOutput=DiscIntNeverNeededParam  ICPrevScaledInput=DiscIntNeverNeededParam
  Fcn1 : Fcn  Expr=Lm*u(2)/(u(1)*Tr+1e-3)
  Gain1 : Gain  Gain=P/2
  Mux1 : Mux  Inputs=2
  Scope : Scope  NumInputPorts=2
  theta : Outport
  wires:
  Discrete-Time Integrator/1 -> theta/1, Scope/1
  iq/1 -> Mux1/2
  wm/1 -> Gain1/1
  Add/1 -> Discrete-Time Integrator/1, Scope/2
  Mux1/1 -> Fcn1/1
  Fcn1/1 -> Add/1
  Phir/1 -> Mux1/1
  Gain1/1 -> Add/2

== system Torque Vectoring and Ackerman Model/Left Motor/FOC1/Vd ==
  Phir* : Inport
  id : Inport  Port=2
  Current PI : pid_lib/PID Controller  Controller=PI  Form=Parallel  TimeDomain=Discrete-time  UseExternalTs=off  SampleTime=Ts  IntegratorMethod=Forward Euler  FilterMethod=Forward Euler  ControllerParametersSource=internal  P=Kp  I=Ki  D=0  UseFilter=on  N=100  TunerSelectOption=Transfer Function Based (PID Tuner App)  InitialConditionSource=internal  InitialConditionForIntegrator=0  InitialConditionForFilter=0  DifferentiatorICPrevScaledInput=0  ExternalReset=none  TrackingMode=off  Kt=1  LimitOutput=on  SatLimitsSource=internal  UpperSaturationLimit=VDC  LowerSaturationLimit=-VDC/2  LinearizeAsGain=off  AntiWindupMode=clamping  Kb=1  POutMin=[]  POutMax=[]  IOutMin=[]  IOutMax=[]  DOutMin=[]  DOutMax=[]  NOutMin=[]  NOutMax=[]  SumOutMin=[]  SumOutMax=[]  SaturationOutMin=[]  SaturationOutMax=[]  PParamMin=[]  PParamMax=[]  IParamMin=[]  IParamMax=[]  DParamMin=[]  DParamMax=[]  NParamMin=[]  NParamMax=[]  KbParamMin=[]  KbParamMax=[]  KtParamMin=[]  KtParamMax=[]  KbOutMin=[]  KbOutMax=[]  KtOutMin=[]  KtOutMax=[]  IntegratorOutMin=[]  IntegratorOutMax=[]  FilterOutMin=[]  FilterOutMax=[]  SumI1OutMin=[]  SumI1OutMax=[]  SumI2OutMin=[]  SumI2OutMax=[]  SumI3OutMin=[]  SumI3OutMax=[]  SumI4OutMin=[]  SumI4OutMax=[]  SumDOutMin=[]  SumDOutMax=[]  DifferentiatorOutMin=[]  DifferentiatorOutMax=[]  FilterDiffOutCoefMin=[]  FilterDiffOutCoefMax=[]  ReciprocalOutMin=[]  ReciprocalOutMax=[]  SumDenOutMin=[]  SumDenOutMax=[]  SumNumOutMin=[]  SumNumOutMax=[]  DivideOutMin=[]  DivideOutMax=[]  UdiffTsProdOutMin=[]  UdiffTsProdOutMax=[]  NTsProdOutMin=[]  NTsProdOutMax=[]  UintegralTsProdOutMin=[]  UintegralTsProdOutMax=[]  UngainTsProdOutMin=[]  UngainTsProdOutMax=[]  IntegratorContinuousStateAttributes=''  IntegratorStateMustResolveToSignalObject=off  IntegratorRTWStateStorageClass=Auto  FilterContinuousStateAttributes=''  FilterStateMustResolveToSignalObject=off  FilterRTWStateStorageClass=Auto  ParallelPVariant=InternalParameters  IdealPVariant=Disabled  IVariant=InternalParameters  DVariant=Disabled  IntegratorVariant=Discrete  SatVariant=Enabled  AWVariant=DiscClampingParallel  PCopyVariant=Disabled  TRVariant=Disabled  FdbkBlocksVariant=Forward  IdealPFdbkVariant=Disabled  SatFdbkVariant=Disabled  DerivativeFilterVariant=Disabled  NVariant=Disabled  NCopyVariant=Disabled_SignalSpec  FilterICVariant=Disabled  IntegratorICVariant=InternalICs  ExternalResetVariant=Disabled  TRSumVariant=Passthrough  SumFdbkVariant=Disabled  SumVariant=Sum_PI  TsampFilterVariant=InternalTs  TsampNgainVariant=Passthrough  TsampIntegralVariant=Passthrough  ExternalSaturationOutDataTypeStr=Inherit: Same as second input
  Gain : Gain  Gain=1/Lm
  Scope : Scope
  Sum2 : Sum  Inputs=|+-
  Vd : Outport
  tag scope: IdrefL=global
  wires:
  Current PI/1 -> Vd/1
  Sum2/1 -> Current PI/1
  id/1 -> Sum2/2
  Phir*/1 -> Gain/1
  Gain/1 -> Sum2/1, Scope/1, [IdrefL]

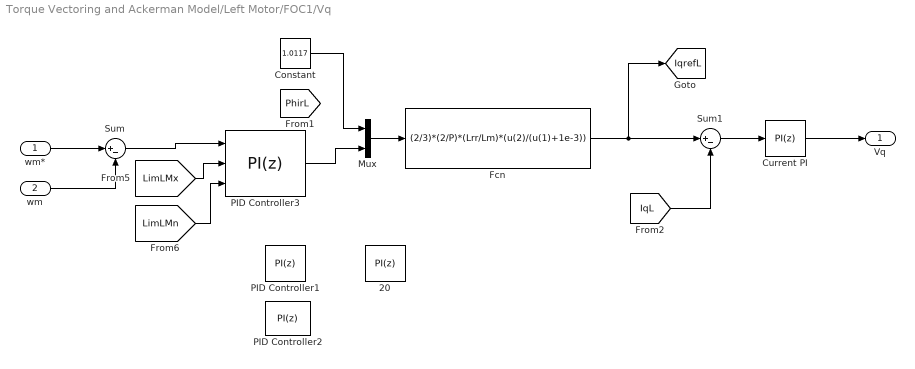
== system Torque Vectoring and Ackerman Model/Left Motor/FOC1/Vq ==
  wm* : Inport
  wm : Inport  Port=2
  20 : pid_lib/PID Controller  Controller=PI  Form=Parallel  TimeDomain=Discrete-time  UseExternalTs=off  SampleTime=-1  IntegratorMethod=Forward Euler  FilterMethod=Forward Euler  ControllerParametersSource=internal  P=152.4390244  I=9295.062463  D=0  UseFilter=on  N=100  TunerSelectOption=Transfer Function Based (PID Tuner App)  InitialConditionSource=internal  InitialConditionForIntegrator=0  InitialConditionForFilter=0  DifferentiatorICPrevScaledInput=0  ExternalReset=none  TrackingMode=off  Kt=1  LimitOutput=on  SatLimitsSource=internal  UpperSaturationLimit=960  LowerSaturationLimit=-960  LinearizeAsGain=off  AntiWindupMode=clamping  Kb=1  POutMin=[]  POutMax=[]  IOutMin=[]  IOutMax=[]  DOutMin=[]  DOutMax=[]  NOutMin=[]  NOutMax=[]  SumOutMin=[]  SumOutMax=[]  SaturationOutMin=[]  SaturationOutMax=[]  PParamMin=[]  PParamMax=[]  IParamMin=[]  IParamMax=[]  DParamMin=[]  DParamMax=[]  NParamMin=[]  NParamMax=[]  KbParamMin=[]  KbParamMax=[]  KtParamMin=[]  KtParamMax=[]  KbOutMin=[]  KbOutMax=[]  KtOutMin=[]  KtOutMax=[]  IntegratorOutMin=[]  IntegratorOutMax=[]  FilterOutMin=[]  FilterOutMax=[]  SumI1OutMin=[]  SumI1OutMax=[]  SumI2OutMin=[]  SumI2OutMax=[]  SumI3OutMin=[]  SumI3OutMax=[]  SumI4OutMin=[]  SumI4OutMax=[]  SumDOutMin=[]  SumDOutMax=[]  DifferentiatorOutMin=[]  DifferentiatorOutMax=[]  FilterDiffOutCoefMin=[]  FilterDiffOutCoefMax=[]  ReciprocalOutMin=[]  ReciprocalOutMax=[]  SumDenOutMin=[]  SumDenOutMax=[]  SumNumOutMin=[]  SumNumOutMax=[]  DivideOutMin=[]  DivideOutMax=[]  UdiffTsProdOutMin=[]  UdiffTsProdOutMax=[]  NTsProdOutMin=[]  NTsProdOutMax=[]  UintegralTsProdOutMin=[]  UintegralTsProdOutMax=[]  UngainTsProdOutMin=[]  UngainTsProdOutMax=[]  IntegratorContinuousStateAttributes=''  IntegratorStateMustResolveToSignalObject=off  IntegratorRTWStateStorageClass=Auto  FilterContinuousStateAttributes=''  FilterStateMustResolveToSignalObject=off  FilterRTWStateStorageClass=Auto  ParallelPVariant=InternalParameters  IdealPVariant=Disabled  IVariant=InternalParameters  DVariant=Disabled  IntegratorVariant=Discrete  SatVariant=Enabled  AWVariant=DiscClampingParallel  PCopyVariant=Disabled  TRVariant=Disabled  FdbkBlocksVariant=Forward  IdealPFdbkVariant=Disabled  SatFdbkVariant=Disabled  DerivativeFilterVariant=Disabled  NVariant=Disabled  NCopyVariant=Disabled_SignalSpec  FilterICVariant=Disabled  IntegratorICVariant=InternalICs  ExternalResetVariant=Disabled  TRSumVariant=Passthrough  SumFdbkVariant=Disabled  SumVariant=Sum_PI  TsampFilterVariant=InternalTs  TsampNgainVariant=Passthrough  TsampIntegralVariant=Passthrough  ExternalSaturationOutDataTypeStr=Inherit: Same as second input
  Constant : Constant  Value=1.0117
  Current PI : pid_lib/PID Controller  Controller=PI  Form=Parallel  TimeDomain=Discrete-time  UseExternalTs=off  SampleTime=Ts  IntegratorMethod=Forward Euler  FilterMethod=Forward Euler  ControllerParametersSource=internal  P=Kp  I=Ki  D=0  UseFilter=on  N=100  TunerSelectOption=Transfer Function Based (PID Tuner App)  InitialConditionSource=internal  InitialConditionForIntegrator=0  InitialConditionForFilter=0  DifferentiatorICPrevScaledInput=0  ExternalReset=none  TrackingMode=off  Kt=1  LimitOutput=on  SatLimitsSource=internal  UpperSaturationLimit=VDC/sqrt(3)  LowerSaturationLimit=-VDC/sqrt(3)  LinearizeAsGain=off  AntiWindupMode=clamping  Kb=1  POutMin=[]  POutMax=[]  IOutMin=[]  IOutMax=[]  DOutMin=[]  DOutMax=[]  NOutMin=[]  NOutMax=[]  SumOutMin=[]  SumOutMax=[]  SaturationOutMin=[]  SaturationOutMax=[]  PParamMin=[]  PParamMax=[]  IParamMin=[]  IParamMax=[]  DParamMin=[]  DParamMax=[]  NParamMin=[]  NParamMax=[]  KbParamMin=[]  KbParamMax=[]  KtParamMin=[]  KtParamMax=[]  KbOutMin=[]  KbOutMax=[]  KtOutMin=[]  KtOutMax=[]  IntegratorOutMin=[]  IntegratorOutMax=[]  FilterOutMin=[]  FilterOutMax=[]  SumI1OutMin=[]  SumI1OutMax=[]  SumI2OutMin=[]  SumI2OutMax=[]  SumI3OutMin=[]  SumI3OutMax=[]  SumI4OutMin=[]  SumI4OutMax=[]  SumDOutMin=[]  SumDOutMax=[]  DifferentiatorOutMin=[]  DifferentiatorOutMax=[]  FilterDiffOutCoefMin=[]  FilterDiffOutCoefMax=[]  ReciprocalOutMin=[]  ReciprocalOutMax=[]  SumDenOutMin=[]  SumDenOutMax=[]  SumNumOutMin=[]  SumNumOutMax=[]  DivideOutMin=[]  DivideOutMax=[]  UdiffTsProdOutMin=[]  UdiffTsProdOutMax=[]  NTsProdOutMin=[]  NTsProdOutMax=[]  UintegralTsProdOutMin=[]  UintegralTsProdOutMax=[]  UngainTsProdOutMin=[]  UngainTsProdOutMax=[]  IntegratorContinuousStateAttributes=''  IntegratorStateMustResolveToSignalObject=off  IntegratorRTWStateStorageClass=Auto  FilterContinuousStateAttributes=''  FilterStateMustResolveToSignalObject=off  FilterRTWStateStorageClass=Auto  ParallelPVariant=InternalParameters  IdealPVariant=Disabled  IVariant=InternalParameters  DVariant=Disabled  IntegratorVariant=Discrete  SatVariant=Enabled  AWVariant=DiscClampingParallel  PCopyVariant=Disabled  TRVariant=Disabled  FdbkBlocksVariant=Forward  IdealPFdbkVariant=Disabled  SatFdbkVariant=Disabled  DerivativeFilterVariant=Disabled  NVariant=Disabled  NCopyVariant=Disabled_SignalSpec  FilterICVariant=Disabled  IntegratorICVariant=InternalICs  ExternalResetVariant=Disabled  TRSumVariant=Passthrough  SumFdbkVariant=Disabled  SumVariant=Sum_PI  TsampFilterVariant=InternalTs  TsampNgainVariant=Passthrough  TsampIntegralVariant=Passthrough  ExternalSaturationOutDataTypeStr=Inherit: Same as second input
  Fcn : Fcn  Expr=(2/3)*(2/P)*(Lrr/Lm)*(u(2)/(u(1)+1e-3))
  Mux : Mux  Inputs=2
  PID Controller1 : pid_lib/PID Controller  Controller=PI  Form=Parallel  TimeDomain=Discrete-time  UseExternalTs=off  SampleTime=-1  IntegratorMethod=Forward Euler  FilterMethod=Forward Euler  ControllerParametersSource=internal  P=105.005210798555  I=869.041988278239  D=0  UseFilter=on  N=100  TunerSelectOption=Transfer Function Based (PID Tuner App)  InitialConditionSource=internal  InitialConditionForIntegrator=0  InitialConditionForFilter=0  DifferentiatorICPrevScaledInput=0  ExternalReset=none  TrackingMode=off  Kt=1  LimitOutput=on  SatLimitsSource=internal  UpperSaturationLimit=960  LowerSaturationLimit=-960  LinearizeAsGain=off  AntiWindupMode=clamping  Kb=1  POutMin=[]  POutMax=[]  IOutMin=[]  IOutMax=[]  DOutMin=[]  DOutMax=[]  NOutMin=[]  NOutMax=[]  SumOutMin=[]  SumOutMax=[]  SaturationOutMin=[]  SaturationOutMax=[]  PParamMin=[]  PParamMax=[]  IParamMin=[]  IParamMax=[]  DParamMin=[]  DParamMax=[]  NParamMin=[]  NParamMax=[]  KbParamMin=[]  KbParamMax=[]  KtParamMin=[]  KtParamMax=[]  KbOutMin=[]  KbOutMax=[]  KtOutMin=[]  KtOutMax=[]  IntegratorOutMin=[]  IntegratorOutMax=[]  FilterOutMin=[]  FilterOutMax=[]  SumI1OutMin=[]  SumI1OutMax=[]  SumI2OutMin=[]  SumI2OutMax=[]  SumI3OutMin=[]  SumI3OutMax=[]  SumI4OutMin=[]  SumI4OutMax=[]  SumDOutMin=[]  SumDOutMax=[]  DifferentiatorOutMin=[]  DifferentiatorOutMax=[]  FilterDiffOutCoefMin=[]  FilterDiffOutCoefMax=[]  ReciprocalOutMin=[]  ReciprocalOutMax=[]  SumDenOutMin=[]  SumDenOutMax=[]  SumNumOutMin=[]  SumNumOutMax=[]  DivideOutMin=[]  DivideOutMax=[]  UdiffTsProdOutMin=[]  UdiffTsProdOutMax=[]  NTsProdOutMin=[]  NTsProdOutMax=[]  UintegralTsProdOutMin=[]  UintegralTsProdOutMax=[]  UngainTsProdOutMin=[]  UngainTsProdOutMax=[]  IntegratorContinuousStateAttributes=''  IntegratorStateMustResolveToSignalObject=off  IntegratorRTWStateStorageClass=Auto  FilterContinuousStateAttributes=''  FilterStateMustResolveToSignalObject=off  FilterRTWStateStorageClass=Auto  ParallelPVariant=InternalParameters  IdealPVariant=Disabled  IVariant=InternalParameters  DVariant=Disabled  IntegratorVariant=Discrete  SatVariant=Enabled  AWVariant=DiscClampingParallel  PCopyVariant=Disabled  TRVariant=Disabled  FdbkBlocksVariant=Forward  IdealPFdbkVariant=Disabled  SatFdbkVariant=Disabled  DerivativeFilterVariant=Disabled  NVariant=Disabled  NCopyVariant=Disabled_SignalSpec  FilterICVariant=Disabled  IntegratorICVariant=InternalICs  ExternalResetVariant=Disabled  TRSumVariant=Passthrough  SumFdbkVariant=Disabled  SumVariant=Sum_PI  TsampFilterVariant=InternalTs  TsampNgainVariant=Passthrough  TsampIntegralVariant=Passthrough  ExternalSaturationOutDataTypeStr=Inherit: Same as second input
  PID Controller2 : pid_lib/PID Controller  Controller=PI  Form=Parallel  TimeDomain=Discrete-time  UseExternalTs=off  SampleTime=-1  IntegratorMethod=Forward Euler  FilterMethod=Forward Euler  ControllerParametersSource=internal  P=287.619  I=35430.839  D=0  UseFilter=on  N=100  TunerSelectOption=Transfer Function Based (PID Tuner App)  InitialConditionSource=internal  InitialConditionForIntegrator=0  InitialConditionForFilter=0  DifferentiatorICPrevScaledInput=0  ExternalReset=none  TrackingMode=off  Kt=1  LimitOutput=on  SatLimitsSource=internal  UpperSaturationLimit=960  LowerSaturationLimit=-960  LinearizeAsGain=off  AntiWindupMode=clamping  Kb=1  POutMin=[]  POutMax=[]  IOutMin=[]  IOutMax=[]  DOutMin=[]  DOutMax=[]  NOutMin=[]  NOutMax=[]  SumOutMin=[]  SumOutMax=[]  SaturationOutMin=[]  SaturationOutMax=[]  PParamMin=[]  PParamMax=[]  IParamMin=[]  IParamMax=[]  DParamMin=[]  DParamMax=[]  NParamMin=[]  NParamMax=[]  KbParamMin=[]  KbParamMax=[]  KtParamMin=[]  KtParamMax=[]  KbOutMin=[]  KbOutMax=[]  KtOutMin=[]  KtOutMax=[]  IntegratorOutMin=[]  IntegratorOutMax=[]  FilterOutMin=[]  FilterOutMax=[]  SumI1OutMin=[]  SumI1OutMax=[]  SumI2OutMin=[]  SumI2OutMax=[]  SumI3OutMin=[]  SumI3OutMax=[]  SumI4OutMin=[]  SumI4OutMax=[]  SumDOutMin=[]  SumDOutMax=[]  DifferentiatorOutMin=[]  DifferentiatorOutMax=[]  FilterDiffOutCoefMin=[]  FilterDiffOutCoefMax=[]  ReciprocalOutMin=[]  ReciprocalOutMax=[]  SumDenOutMin=[]  SumDenOutMax=[]  SumNumOutMin=[]  SumNumOutMax=[]  DivideOutMin=[]  DivideOutMax=[]  UdiffTsProdOutMin=[]  UdiffTsProdOutMax=[]  NTsProdOutMin=[]  NTsProdOutMax=[]  UintegralTsProdOutMin=[]  UintegralTsProdOutMax=[]  UngainTsProdOutMin=[]  UngainTsProdOutMax=[]  IntegratorContinuousStateAttributes=''  IntegratorStateMustResolveToSignalObject=off  IntegratorRTWStateStorageClass=Auto  FilterContinuousStateAttributes=''  FilterStateMustResolveToSignalObject=off  FilterRTWStateStorageClass=Auto  ParallelPVariant=InternalParameters  IdealPVariant=Disabled  IVariant=InternalParameters  DVariant=Disabled  IntegratorVariant=Discrete  SatVariant=Enabled  AWVariant=DiscClampingParallel  PCopyVariant=Disabled  TRVariant=Disabled  FdbkBlocksVariant=Forward  IdealPFdbkVariant=Disabled  SatFdbkVariant=Disabled  DerivativeFilterVariant=Disabled  NVariant=Disabled  NCopyVariant=Disabled_SignalSpec  FilterICVariant=Disabled  IntegratorICVariant=InternalICs  ExternalResetVariant=Disabled  TRSumVariant=Passthrough  SumFdbkVariant=Disabled  SumVariant=Sum_PI  TsampFilterVariant=InternalTs  TsampNgainVariant=Passthrough  TsampIntegralVariant=Passthrough  ExternalSaturationOutDataTypeStr=Inherit: Same as second input
  PID Controller3 : pid_lib/PID Controller  Controller=PI  Form=Parallel  TimeDomain=Discrete-time  UseExternalTs=off  SampleTime=-1  IntegratorMethod=Forward Euler  FilterMethod=Forward Euler  ControllerParametersSource=internal  P=152.4390244  I=9295.062463  D=0  UseFilter=on  N=100  TunerSelectOption=Transfer Function Based (PID Tuner App)  InitialConditionSource=internal  InitialConditionForIntegrator=0  InitialConditionForFilter=0  DifferentiatorICPrevScaledInput=0  ExternalReset=none  TrackingMode=off  Kt=1  LimitOutput=on  SatLimitsSource=external  UpperSaturationLimit=960  LowerSaturationLimit=-960  LinearizeAsGain=off  AntiWindupMode=clamping  Kb=1  POutMin=[]  POutMax=[]  IOutMin=[]  IOutMax=[]  DOutMin=[]  DOutMax=[]  NOutMin=[]  NOutMax=[]  SumOutMin=[]  SumOutMax=[]  SaturationOutMin=[]  SaturationOutMax=[]  PParamMin=[]  PParamMax=[]  IParamMin=[]  IParamMax=[]  DParamMin=[]  DParamMax=[]  NParamMin=[]  NParamMax=[]  KbParamMin=[]  KbParamMax=[]  KtParamMin=[]  KtParamMax=[]  KbOutMin=[]  KbOutMax=[]  KtOutMin=[]  KtOutMax=[]  IntegratorOutMin=[]  IntegratorOutMax=[]  FilterOutMin=[]  FilterOutMax=[]  SumI1OutMin=[]  SumI1OutMax=[]  SumI2OutMin=[]  SumI2OutMax=[]  SumI3OutMin=[]  SumI3OutMax=[]  SumI4OutMin=[]  SumI4OutMax=[]  SumDOutMin=[]  SumDOutMax=[]  DifferentiatorOutMin=[]  DifferentiatorOutMax=[]  FilterDiffOutCoefMin=[]  FilterDiffOutCoefMax=[]  ReciprocalOutMin=[]  ReciprocalOutMax=[]  SumDenOutMin=[]  SumDenOutMax=[]  SumNumOutMin=[]  SumNumOutMax=[]  DivideOutMin=[]  DivideOutMax=[]  UdiffTsProdOutMin=[]  UdiffTsProdOutMax=[]  NTsProdOutMin=[]  NTsProdOutMax=[]  UintegralTsProdOutMin=[]  UintegralTsProdOutMax=[]  UngainTsProdOutMin=[]  UngainTsProdOutMax=[]  IntegratorContinuousStateAttributes=''  IntegratorStateMustResolveToSignalObject=off  IntegratorRTWStateStorageClass=Auto  FilterContinuousStateAttributes=''  FilterStateMustResolveToSignalObject=off  FilterRTWStateStorageClass=Auto  ParallelPVariant=InternalParameters  IdealPVariant=Disabled  IVariant=InternalParameters  DVariant=Disabled  IntegratorVariant=Discrete  SatVariant=External  AWVariant=DiscClampingParallel  PCopyVariant=Disabled  TRVariant=Disabled  FdbkBlocksVariant=Forward  IdealPFdbkVariant=Disabled  SatFdbkVariant=Disabled  DerivativeFilterVariant=Disabled  NVariant=Disabled  NCopyVariant=Disabled_SignalSpec  FilterICVariant=Disabled  IntegratorICVariant=InternalICs  ExternalResetVariant=Disabled  TRSumVariant=Passthrough  SumFdbkVariant=Disabled  SumVariant=Sum_PI  TsampFilterVariant=InternalTs  TsampNgainVariant=Passthrough  TsampIntegralVariant=Passthrough  ExternalSaturationOutDataTypeStr=Inherit: Same as second input
  Sum : Sum  Inputs=|+-
  Sum1 : Sum  Inputs=|+-
  Vq : Outport
  tag scope: IqrefL=global
  wires:
  Constant/1 -> Mux/1
  Current PI/1 -> Vq/1
  Sum1/1 -> Current PI/1
  Fcn/1 -> [IqrefL], Sum1/1
  [IqL] -> Sum1/2
  wm*/1 -> Sum/1
  Mux/1 -> Fcn/1
  wm/1 -> Sum/2
  Sum/1 -> PID Controller3/1
  PID Controller3/1 -> Mux/2
  [LimLMx] -> PID Controller3/2
  [LimLMn] -> PID Controller3/3

== system Torque Vectoring and Ackerman Model/Right Motor/FOC1/ABC to qd ==
  abc : Inport
  wt : Inport  Port=2
  Demux : Demux  Outputs=3
  Terminator : Terminator
  Unit Delay : UnitDelay  SampleTime=-1  HasFrameUpgradeWarning=on
  Unit Delay1 : UnitDelay  SampleTime=-1  HasFrameUpgradeWarning=on
  abc to dq0 : powerlib_meascontrol/Transformations/abc to dq0  Alignment=90 degrees behind phase A axis
  id : Outport
  iq : Outport  Port=2
  wires:
  Demux/1 -> Unit Delay/1
  Demux/3 -> Terminator/1
  abc to dq0/1 -> Demux/1
  Demux/2 -> Unit Delay1/1
  Unit Delay/1 -> iq/1
  wt/1 -> abc to dq0/2
  Unit Delay1/1 -> id/1
  abc/1 -> abc to dq0/1

== system Torque Vectoring and Ackerman Model/Right Motor/FOC1/Phir calculation ==
  id : Inport
  Transfer Fcn : TransferFcn  Numerator=[Lm]  Denominator=[Tr 1]
  Phir : Outport
  wires:
  Transfer Fcn/1 -> Phir/1
  id/1 -> Transfer Fcn/1

== system Torque Vectoring and Ackerman Model/Right Motor/FOC1/SVPWM ==
  In1 : Inport
  In2 : Inport  Port=2
  Constant1 : Constant  Value=0
  Demux1 : Demux  Outputs=3
  Mux2 : Mux  Inputs=3
  SVPWM Generator (2-Level) : powerlib_meascontrol/Pulse & Signal Generators/SVPWM Generator (2-Level)  InputType=alpha-beta components  SwitchingPattern=Pattern #1  Fc=5000  ParUref=[0.8 -30 50]  Ts=0
      settings: SourceProductBaseCode=PS
  Terminator1 : Terminator
  dq0 to Alpha-Beta-Zero : powerlib_meascontrol/Transformations/dq0 to Alpha-Beta-Zero  Alignment=90 degrees behind phase A axis
      settings: SourceProductBaseCode=PS
  P : Outport
  wires:
  Demux1/2 -> SVPWM Generator (2-Level)/2
  Demux1/3 -> Terminator1/1
  Mux2/1 -> dq0 to Alpha-Beta-Zero/1
  In1/1 -> Mux2/1
  SVPWM Generator (2-Level)/1 -> P/1
  In2/1 -> Mux2/2
  [ThetaR] -> dq0 to Alpha-Beta-Zero/2
  dq0 to Alpha-Beta-Zero/1 -> Demux1/1
  Constant1/1 -> Mux2/3
  Demux1/1 -> SVPWM Generator (2-Level)/1

== system Torque Vectoring and Ackerman Model/Right Motor/FOC1/Theta calulation ==
  Phir : Inport
  iq : Inport  Port=2
  wm : Inport  Port=3
  Add : Sum
  Discrete-Time Integrator : DiscreteIntegrator  SampleTime=Ts  ICPrevOutput=DiscIntNeverNeededParam  ICPrevScaledInput=DiscIntNeverNeededParam
  Fcn1 : Fcn  Expr=Lm*u(2)/(u(1)*Tr+1e-3)
  Gain1 : Gain  Gain=P/2
  Mux1 : Mux  Inputs=2
  Scope : Scope  NumInputPorts=2
  theta : Outport
  wires:
  Gain1/1 -> Add/2
  Phir/1 -> Mux1/1
  Fcn1/1 -> Add/1
  Mux1/1 -> Fcn1/1
  Add/1 -> Scope/2, Discrete-Time Integrator/1
  wm/1 -> Gain1/1
  iq/1 -> Mux1/2
  Discrete-Time Integrator/1 -> Scope/1, theta/1
